simulink model "softarm_plant"  (R2025a)
settings: Solver=ode15s  StartTime=0.0  StopTime=5  RelTol=1e-3
model mask{Bundle=Bundle}
  mask prompts: Bundle "Bundle directory"
PreLoadFcn:
  | softarm_root=fileparts(get_param(bdroot,'FileName'));addpath(softarm_root);addpath(fullfile(softarm_root,'matlab'));
model workspace (MAT data in the model file):
  Bundle = 'examples/generated/pcc_lumped_n2'
undefined symbols (not defined in the file or in its folder): softarm_nq, softarm_p, softarm_x0
settings Model: ParameterArgumentNames=Bundle  Creator=rlwan  LastModifiedBy=rlwan

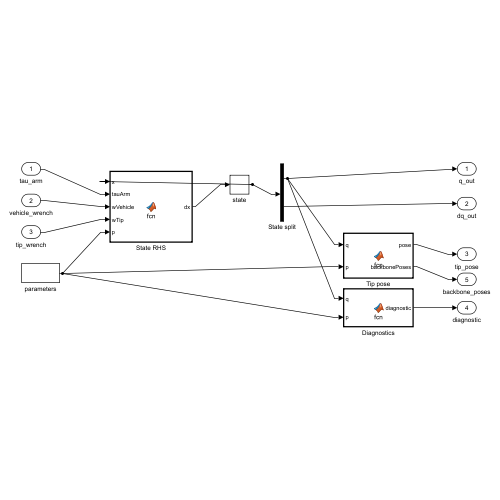
[thumbnail: Simulink's stored preview of the top-level diagram]
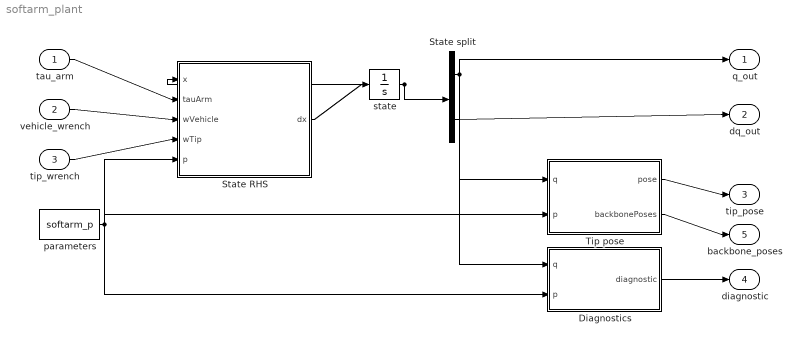
== system softarm_plant ==
  tau_arm : Inport  PortDimensions=softarm_narm
  vehicle_wrench : Inport  Port=2  PortDimensions=6
  tip_wrench : Inport  Port=3  PortDimensions=6
  Diagnostics : MATLAB Function  TreatAsAtomicUnit=on
  State RHS : MATLAB Function  TreatAsAtomicUnit=on
  State split : Demux  Outputs=[softarm_nq softarm_nq]
  Tip pose : MATLAB Function  TreatAsAtomicUnit=on
  parameters : Constant  Value=softarm_p
  state : Integrator  InitialCondition=softarm_x0
  q_out : Outport
  dq_out : Outport  Port=2
  tip_pose : Outport  Port=3
  diagnostic : Outport  Port=4
  backbone_poses : Outport  Port=5
  wires:
  state/1 -> State split/1, State RHS/1(x)
  tau_arm/1 -> State RHS/2(tauArm)
  vehicle_wrench/1 -> State RHS/3(wVehicle)
  tip_wrench/1 -> State RHS/4(wTip)
  parameters/1 -> State RHS/5(p), Tip pose/2(p), Diagnostics/2(p)
  State RHS/1(dx) -> state/1
  State split/1 -> q_out/1, Tip pose/1(q), Diagnostics/1(q)
  State split/2 -> dq_out/1
  Tip pose/1(pose) -> tip_pose/1
  Diagnostics/1(diagnostic) -> diagnostic/1
  Tip pose/2(backbonePoses) -> backbone_poses/1

== matlab function softarm_plant/Tip pose ==
  data: q input; pose output; p input; backbonePoses output
function [pose,backbonePoses] = fcn(q,p)
%#codegen
H=softarm_kinematics(q,p); pose=reshape(H(:,:,end),16,1); backbonePoses=H(:);
end

== matlab function softarm_plant/State RHS ==
  data: x input; dx output; tauArm input; wVehicle input; wTip input; p input
function dx = fcn(x,tauArm,wVehicle,wTip,p)
%#codegen
dx = softarm_state_rhs(x,tauArm,wVehicle,wTip,p);
end

== matlab function softarm_plant/Diagnostics ==
  data: q input; diagnostic output; p input
function diagnostic = fcn(q,p)
%#codegen
diagnostic=rcond(softarm_mass(q,p));
end
